simulink model "ZAD1_2_ObiektARMAX"  (R2018a)
settings: Solver=FixedStepDiscrete  StartTime=0.0  StopTime=Tend  FixedStep=Tp  RelTol=1e-3  EnableMultiTasking=on
values from neighbouring files (symbols this model uses):
  c10 = 0    [ZAD1_1_skrypt.m]    (also in ZAD1_2_skrypt.m = 0.7; ZAD2_1_skrypt.m = 0.7)
  fu = 0.2    [ZAD1_1_skrypt.m]    (also in ZAD1_2_skrypt.m; ZAD2_1_skrypt.m)
  Td = 1500    [ZAD1_1_skrypt.m]    (also in ZAD1_2_skrypt.m; ZAD2_1_skrypt.m = 300)
  Tp = 0.1    [ZAD1_1_skrypt.m]    (also in ZAD1_2_skrypt.m; ZAD2_1_skrypt.m)
libraries: simulink x1
settings Model: Creator=szymon  LastModifiedBy=szymon
settings DataIOCC: LimitDataPoints=on  SaveFormat=Array
settings OptimizationCC: InitFltsAndDblsToZero=on  LifeSpan=inf
settings DebuggingCC: SaveWithParameterizedLinksMsg=none  UnderspecifiedInitializationDetection=Classic  MergeDetectMultiDrivingBlocksExec=none  SignalResolutionControl=TryResolveAllWithWarning  SolverPrmCheckMsg=warning  MultiTaskDSMMsg=warning  MultiTaskCondExecSysMsg=none  FcnCallInpInsideContextMsg=warning  SFUnexpectedBacktrackingDiag=warning  SFNoUnconditionalDefaultTransitionDiag=warning  SFExecutionAtInitializationDiag=none
settings HardwareCC: ProdBitPerPointer=32  ProdBitPerSizeT=32  ProdBitPerPtrDiffT=32  ProdLargestAtomicFloat=None  ProdIntDivRoundTo=Undefined  ProdEndianess=Unspecified  ProdWordSize=32  ProdHWDeviceType=32-bit Generic
settings ModelReferenceCC: PropagateSignalLabelsOutOfModel=off
settings CodeAppCC: StateflowObjectComments=on
settings GRTTargetCC: TargetFcnLib=ansi_tfl_tmw.mat  TargetLangStandard=C89/C90 (ANSI)  CombineOutputUpdateFcns=off  GRTInterface=on
settings ConfigComp: CovMetricSettings=dw  CovHtmlReporting=on  CovSaveCumulativeToWorkspaceVar=on  CovSaveSingleToWorkspaceVar=on  CovExternalEMLEnable=off

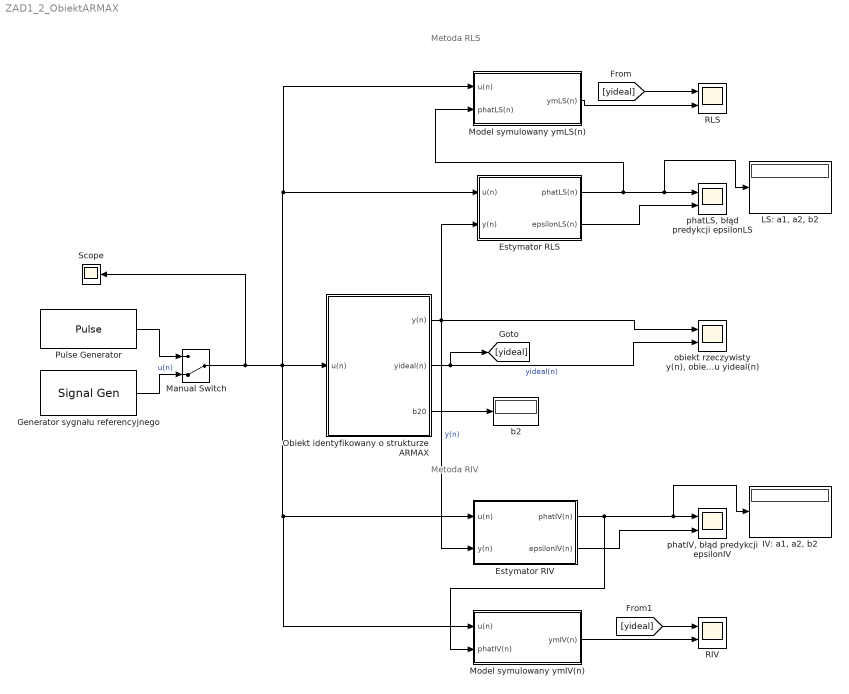
== system ZAD1_2_ObiektARMAX ==
  note: Metoda RLS
  note: Metoda RIV
  Estymator RIV : Subsystem
  Estymator RLS : Subsystem
  Generator sygnału referencyjnego : SignalGenerator  WaveForm=square  Frequency=fu
  "IV: a1, a2, b2" : Display
  "LS: a1, a2, b2" : Display
  Manual Switch : ManualSwitch  CurrentSetting=0
  Model symulowany ymIV(n) : Subsystem
  Model symulowany ymLS(n) : Subsystem
  Obiekt identyfikowany o strukturze ARMAX : Subsystem
  Pulse Generator : DiscretePulseGenerator  PulseType=Time based  Period=5  PulseWidth=50
  RIV : Scope  NumInputPorts=2
  RLS : Scope  NumInputPorts=2
  Scope : Scope
  b2 : Display
  "obiekt rzeczywisty y(n), obiekt rzeczywisty bez szumu yideal(n)" : Scope  NumInputPorts=2
  "phatIV, błąd predykcji epsilonIV" : Scope  NumInputPorts=2
  "phatLS, błąd predykcji epsilonLS" : Scope  NumInputPorts=2
  wires:
  Obiekt identyfikowany o strukturze ARMAX/1(y(n)) -> Estymator RLS/2(y(n)), "obiekt rzeczywisty y(n), obiekt rzeczywisty bez szumu yideal(n)"/1, Estymator RIV/2(y(n))  "y(n)"
  Estymator RLS/1(phatLS(n)) -> Model symulowany ymLS(n)/2(phatLS(n)), "LS: a1, a2, b2"/1, "phatLS, błąd predykcji epsilonLS"/1
  Estymator RLS/2(epsilonLS(n)) -> "phatLS, błąd predykcji epsilonLS"/2
  [yideal] -> RLS/1
  Model symulowany ymLS(n)/1(ymLS(n)) -> RLS/2
  Obiekt identyfikowany o strukturze ARMAX/2(yideal(n)) -> [yideal], "obiekt rzeczywisty y(n), obiekt rzeczywisty bez szumu yideal(n)"/2  "yideal(n)"
  Estymator RIV/1(phatIV(n)) -> Model symulowany ymIV(n)/2(phatIV(n)), "IV: a1, a2, b2"/1, "phatIV, błąd predykcji epsilonIV"/1
  Estymator RIV/2(epsilonIV(n)) -> "phatIV, błąd predykcji epsilonIV"/2
  [yideal] -> RIV/1
  Model symulowany ymIV(n)/1(ymIV(n)) -> RIV/2
  Pulse Generator/1 -> Manual Switch/1
  Manual Switch/1 -> Scope/1, Model symulowany ymIV(n)/1(u(n)), Estymator RIV/1(u(n)), Model symulowany ymLS(n)/1(u(n)), Estymator RLS/1(u(n)), Obiekt identyfikowany o strukturze ARMAX/1(u(n))
  Generator sygnału referencyjnego/1 -> Manual Switch/2  "u(n)"
  Obiekt identyfikowany o strukturze ARMAX/3(b20) -> b2/1

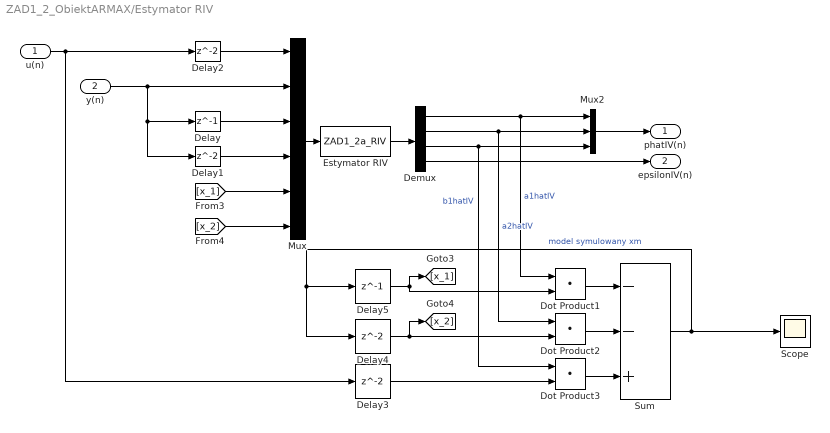
== system ZAD1_2_ObiektARMAX/Estymator RIV ==
  u(n) : Inport
  y(n) : Inport  Port=2
  Delay : Delay  DelayLength=1
  Delay{1..4} (4 alike) : Delay
  Delay5 : Delay  DelayLength=1
  Demux : Demux
  Dot Product1 : DotProduct  InputSameDT=on  OutDataTypeStr=Inherit: Inherit via internal rule
  Dot Product2 : DotProduct  InputSameDT=on  OutDataTypeStr=Inherit: Inherit via internal rule
  Dot Product3 : DotProduct  InputSameDT=on  OutDataTypeStr=Inherit: Inherit via internal rule
  Estymator RIV : MATLABFcn  MATLABFcn=ZAD1_2a_RIV
  Mux : Mux  Inputs=6
  Mux2 : Mux  Inputs=3
  Scope : Scope
  Sum : Sum  Inputs=--+
  phatIV(n) : Outport
  epsilonIV(n) : Outport  Port=2
  wires:
  Estymator RIV/1 -> Demux/1
  Delay2/1 -> Mux/1
  y(n)/1 -> Delay1/1, Delay/1, Mux/2
  Delay/1 -> Mux/3
  Delay1/1 -> Mux/4
  Mux/1 -> Estymator RIV/1
  Demux/4 -> epsilonIV(n)/1
  Mux2/1 -> phatIV(n)/1
  [x_1] -> Mux/5
  [x_2] -> Mux/6
  Demux/1 -> Dot Product1/1, Mux2/1  "a1hatIV"
  Delay3/1 -> Dot Product3/2
  Demux/2 -> Dot Product2/1, Mux2/2  "a2hatIV"
  Delay4/1 -> [x_2], Dot Product2/2
  Demux/3 -> Dot Product3/1, Mux2/3  "b1hatIV"
  Dot Product1/1 -> Sum/1
  u(n)/1 -> Delay3/1, Delay2/1
  Delay5/1 -> Dot Product1/2, [x_1]
  Dot Product2/1 -> Sum/2
  Sum/1 -> Scope/1, Delay4/1, Delay5/1  "model symulowany xm"
  Dot Product3/1 -> Sum/3

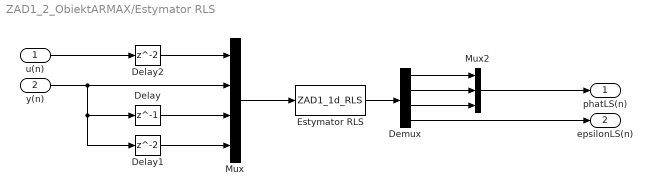
== system ZAD1_2_ObiektARMAX/Estymator RLS ==
  u(n) : Inport
  y(n) : Inport  Port=2
  Delay : Delay  DelayLength=1
  Delay1 : Delay
  Delay2 : Delay
  Demux : Demux
  Estymator RLS : MATLABFcn  MATLABFcn=ZAD1_1d_RLS
  Mux : Mux
  Mux2 : Mux  Inputs=3
  phatLS(n) : Outport
  epsilonLS(n) : Outport  Port=2
  wires:
  Estymator RLS/1 -> Demux/1
  u(n)/1 -> Delay2/1
  Delay2/1 -> Mux/1
  y(n)/1 -> Delay1/1, Delay/1, Mux/2
  Delay/1 -> Mux/3
  Delay1/1 -> Mux/4
  Mux/1 -> Estymator RLS/1
  Demux/4 -> epsilonLS(n)/1
  Demux/1 -> Mux2/1
  Demux/2 -> Mux2/2
  Demux/3 -> Mux2/3
  Mux2/1 -> phatLS(n)/1

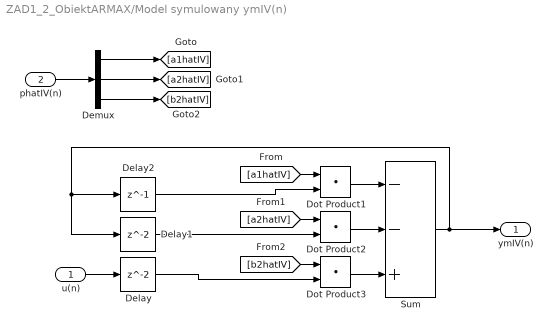
== system ZAD1_2_ObiektARMAX/Model symulowany ymIV(n) ==
  u(n) : Inport
  phatIV(n) : Inport  Port=2
  Delay : Delay
  Delay1 : Delay
  Delay2 : Delay  DelayLength=1
  Demux : Demux  Outputs=3
  Dot Product1 : DotProduct  InputSameDT=on  OutDataTypeStr=Inherit: Inherit via internal rule
  Dot Product2 : DotProduct  InputSameDT=on  OutDataTypeStr=Inherit: Inherit via internal rule
  Dot Product3 : DotProduct  InputSameDT=on  OutDataTypeStr=Inherit: Inherit via internal rule
  Sum : Sum  Inputs=--+
  ymIV(n) : Outport
  wires:
  phatIV(n)/1 -> Demux/1
  u(n)/1 -> Delay/1
  Demux/2 -> [a2hatIV]
  Demux/1 -> [a1hatIV]
  Demux/3 -> [b2hatIV]
  [a1hatIV] -> Dot Product1/1
  Dot Product1/1 -> Sum/1
  Delay2/1 -> Dot Product1/2
  Dot Product2/1 -> Sum/2
  [a2hatIV] -> Dot Product2/1
  [b2hatIV] -> Dot Product3/1
  Dot Product3/1 -> Sum/3
  Delay/1 -> Dot Product3/2
  Sum/1 -> ymIV(n)/1, Delay2/1, Delay1/1
  Delay1/1 -> Dot Product2/2

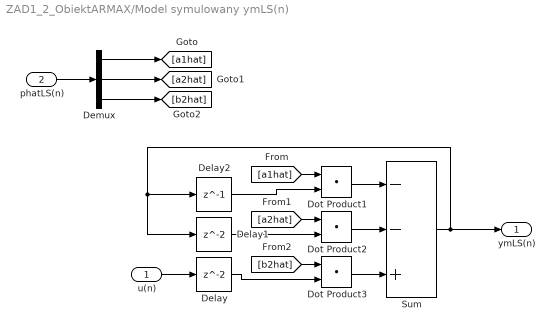
== system ZAD1_2_ObiektARMAX/Model symulowany ymLS(n) ==
  u(n) : Inport
  phatLS(n) : Inport  Port=2
  Delay : Delay
  Delay1 : Delay
  Delay2 : Delay  DelayLength=1
  Demux : Demux  Outputs=3
  Dot Product1 : DotProduct  InputSameDT=on  OutDataTypeStr=Inherit: Inherit via internal rule
  Dot Product2 : DotProduct  InputSameDT=on  OutDataTypeStr=Inherit: Inherit via internal rule
  Dot Product3 : DotProduct  InputSameDT=on  OutDataTypeStr=Inherit: Inherit via internal rule
  Sum : Sum  Inputs=--+
  ymLS(n) : Outport
  wires:
  phatLS(n)/1 -> Demux/1
  u(n)/1 -> Delay/1
  Demux/2 -> [a2hat]
  Demux/1 -> [a1hat]
  Demux/3 -> [b2hat]
  [a1hat] -> Dot Product1/1
  Dot Product1/1 -> Sum/1
  Delay2/1 -> Dot Product1/2
  Dot Product2/1 -> Sum/2
  Delay1/1 -> Dot Product2/2
  [a2hat] -> Dot Product2/1
  [b2hat] -> Dot Product3/1
  Dot Product3/1 -> Sum/3
  Delay/1 -> Dot Product3/2
  Sum/1 -> ymLS(n)/1, Delay2/1, Delay1/1

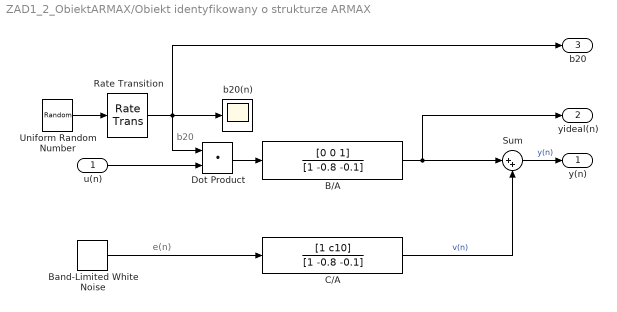
== system ZAD1_2_ObiektARMAX/Obiekt identyfikowany o strukturze ARMAX ==
  note: b20
  note: e(n)
  u(n) : Inport
  B/A : DiscreteFilter  Numerator=[0 0 1]  Denominator=[1 -0.8 -0.1]  SampleTime=Tp
  Band-Limited White Noise : simulink/Sources/Band-Limited White Noise  Cov=[0.001]  Ts=Tp  seed=[23341]
  C/A : DiscreteFilter  Numerator=[1 c10]  Denominator=[1 -0.8 -0.1]  SampleTime=Tp
  Dot Product : DotProduct  InputSameDT=on  OutDataTypeStr=Inherit: Inherit via internal rule
  Rate Transition : RateTransition  InitialCondition=0.5  OutPortSampleTime=Tp
  Sum : Sum  Inputs=|++  SaturateOnIntegerOverflow=on
  Uniform Random Number : UniformRandomNumber  Minimum=0  Maximum=0.5  SampleTime=Td
  b20(n) : Scope
  y(n) : Outport
  yideal(n) : Outport  Port=2
  b20 : Outport  Port=3
  wires:
  C/A/1 -> Sum/2  "v(n)"
  Sum/1 -> y(n)/1  "y(n)"
  Band-Limited White Noise/1 -> C/A/1
  B/A/1 -> yideal(n)/1, Sum/1
  u(n)/1 -> Dot Product/2
  Dot Product/1 -> B/A/1
  Uniform Random Number/1 -> Rate Transition/1
  Rate Transition/1 -> Dot Product/1, b20(n)/1, b20/1
